simulink model "plant"  (R2022b)
settings: Solver=VariableStepAuto  StartTime=0.0  StopTime=20.0  RelTol=1e-3
settings Model: Creator=KHods  LastModifiedBy=KHods

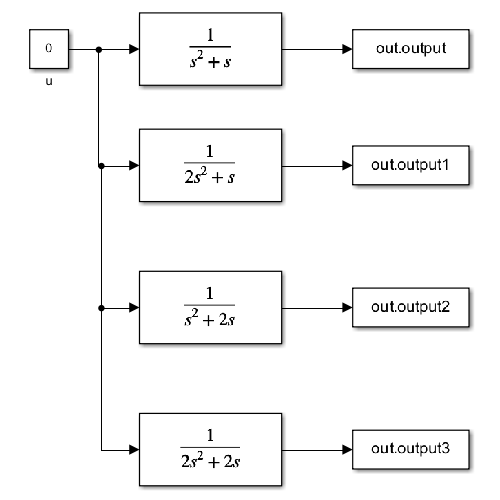
[thumbnail: Simulink's stored preview of the top-level diagram]
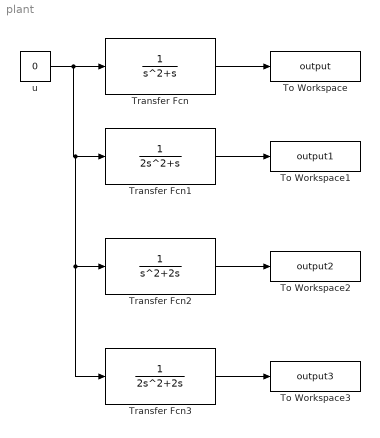
== system plant ==
  To Workspace : ToWorkspace  VariableName=output  SampleTime=-1
      settings: Save2DSignal=2-D array (concatenate along first dimension)
  To Workspace1 : ToWorkspace  VariableName=output1  SampleTime=-1
      settings: Save2DSignal=2-D array (concatenate along first dimension)
  To Workspace2 : ToWorkspace  VariableName=output2  SampleTime=-1
      settings: Save2DSignal=2-D array (concatenate along first dimension)
  To Workspace3 : ToWorkspace  VariableName=output3  SampleTime=-1
      settings: Save2DSignal=2-D array (concatenate along first dimension)
  Transfer Fcn : TransferFcn  Denominator=[1 1 0]
  Transfer Fcn1 : TransferFcn  Denominator=[2 1 0]
  Transfer Fcn2 : TransferFcn  Denominator=[1 2 0]
  Transfer Fcn3 : TransferFcn  Denominator=[2 2 0]
  u : Constant  Value=0
  wires:
  u/1 -> Transfer Fcn3/1, Transfer Fcn2/1, Transfer Fcn1/1, Transfer Fcn/1
  Transfer Fcn/1 -> To Workspace/1
  Transfer Fcn1/1 -> To Workspace1/1
  Transfer Fcn2/1 -> To Workspace2/1
  Transfer Fcn3/1 -> To Workspace3/1
